simulink model "Mfunct2"  (R2020b)
settings: Solver=VariableStepAuto  StartTime=0.0  StopTime=10.0  RelTol=1e-3
libraries: simulink x1
settings Model: Creator=cesar  LastModifiedBy=cesar

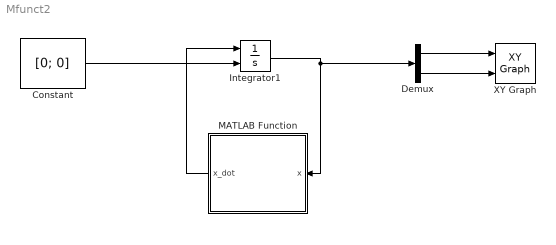
== system Mfunct2 ==
  Constant : Constant  Value=[0; 0]
  Demux : Demux  Outputs=2
  Integrator1 : Integrator  InitialConditionSource=external
  MATLAB Function : MATLAB Function  TreatAsAtomicUnit=on
  XY Graph : simulink/Sinks/XY Graph  xmin=-1  xmax=1  ymin=-1  ymax=1  st=-1
  wires:
  Integrator1/1 -> Demux/1, MATLAB Function/1(x)
  MATLAB Function/1(x_dot) -> Integrator1/1
  Constant/1 -> Integrator1/2
  Demux/1 -> XY Graph/1
  Demux/2 -> XY Graph/2

== matlab function Mfunct2/MATLAB Function ==
  data: x input; x_dot output
function x_dot = fcn(x)

x1_dot = x2;
x2_dot = -x1;

x_dot = [x1_dot; x2_dot];

x = [x1; x2];
